simulink model "Model1"  (R2024b)
settings: Solver=ode8  StartTime=0.0  StopTime=simT  FixedStep=Ts  RelTol=1e-3
values from neighbouring files (symbols this model uses):
  C = 1    [HHparameters.m]
  EK = -12    [HHparameters.m]
  EL = 10.613    [HHparameters.m]
  ENa = 115    [HHparameters.m]
  gbar_K = 36    [HHparameters.m]
  gbar_Na = 120    [HHparameters.m]
  gL = 0.3    [HHparameters.m]
  minf0 = alpham0/(alpham0+betam0)    [HHparameters.m]
settings Model: LastModifiedBy=Matth

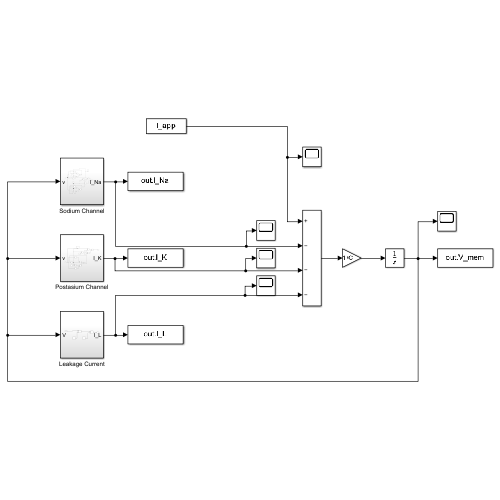
[thumbnail: Simulink's stored preview of the top-level diagram]
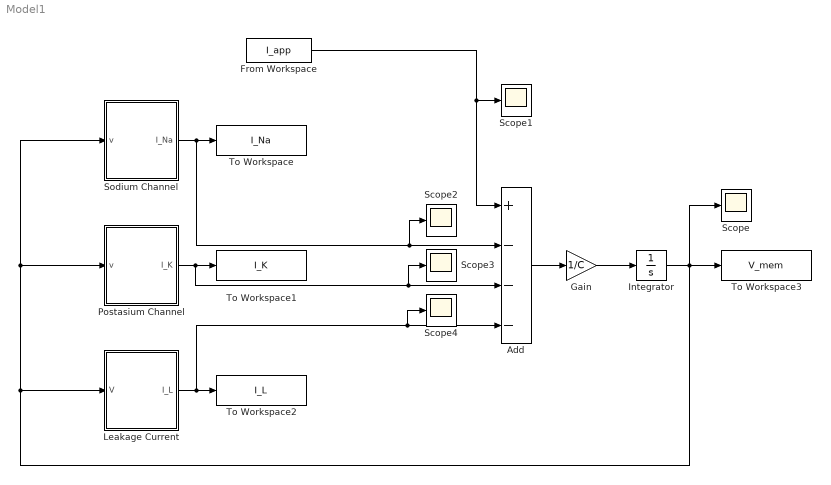
== system Model1 ==
  Add : Sum  Inputs=+---
  From Workspace : FromWorkspace  VariableName=I_app
  Gain : Gain  Gain=1/C
  Integrator : Integrator  InitialCondition=minf0
  Leakage Current : Subsystem
  Postasium Channel : Subsystem
  Scope{,1..4} (5 alike) : Scope
  Sodium Channel : Subsystem
  To Workspace : ToWorkspace  VariableName=I_Na  SampleTime=-1
  To Workspace1 : ToWorkspace  VariableName=I_K  SampleTime=-1
  To Workspace2 : ToWorkspace  VariableName=I_L  SampleTime=-1
  To Workspace3 : ToWorkspace  VariableName=V_mem  SampleTime=-1
  wires:
  Sodium Channel/1(I_Na) -> To Workspace/1, Scope2/1, Add/2
  Gain/1 -> Integrator/1
  Integrator/1 -> To Workspace3/1, Sodium Channel/1(v), Postasium Channel/1(v), Leakage Current/1(V), Scope/1
  Add/1 -> Gain/1
  Postasium Channel/1(I_K) -> To Workspace1/1, Add/3, Scope3/1
  Leakage Current/1(I_L) -> Scope4/1, Add/4, To Workspace2/1
  From Workspace/1 -> Scope1/1, Add/1

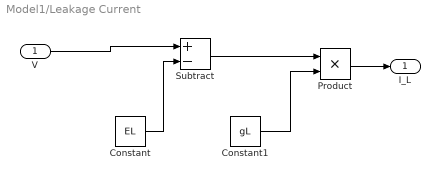
== system Model1/Leakage Current ==
  V : Inport
  Constant : Constant  Value=EL
  Constant1 : Constant  Value=gL
  Product : Product
  Subtract : Sum  Inputs=+-
  I_L : Outport
  wires:
  Constant1/1 -> Product/2
  Constant/1 -> Subtract/2
  V/1 -> Subtract/1
  Subtract/1 -> Product/1
  Product/1 -> I_L/1

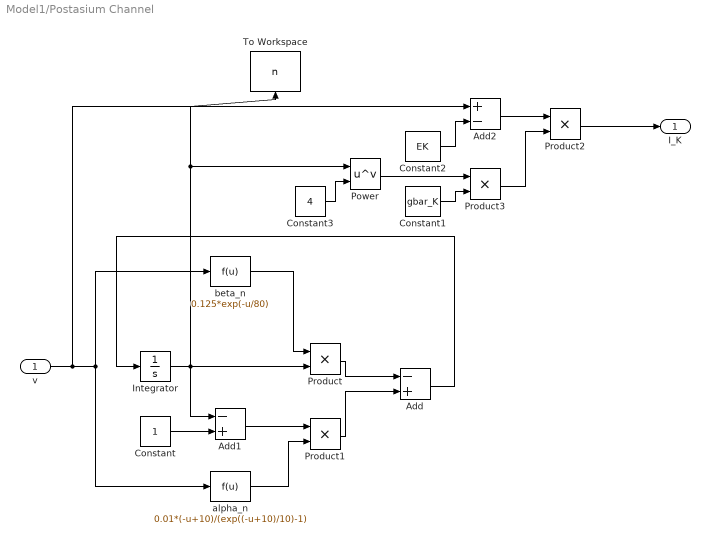
== system Model1/Postasium Channel ==
  v : Inport
  Add : Sum  Inputs=-+
  Add1 : Sum  Inputs=-+
  Add2 : Sum  Inputs=+-
  Constant : Constant
  Constant1 : Constant  Value=gbar_K
  Constant2 : Constant  Value=EK
  Constant3 : Constant  Value=4
  Integrator : Integrator  InitialCondition=0.1/(exp(1)-1)/(0.1/(exp(1)-1)+0.125)
  Power : Math  Operator=pow
  Product{,1..3} (4 alike) : Product
  To Workspace : ToWorkspace  VariableName=n  SaveFormat=Timeseries  SampleTime=-1
  alpha_n : Fcn  Expr=0.01*(-u+10)/(exp((-u+10)/10)-1)
  beta_n : Fcn  Expr=0.125*exp(-u/80)
  I_K : Outport
  wires:
  beta_n/1 -> Product/1
  Product/1 -> Add/1
  Product1/1 -> Add/2
  Add1/1 -> Product1/1
  Constant/1 -> Add1/2
  Add/1 -> Integrator/1
  Integrator/1 -> Product/2, Power/1, To Workspace/1, Add1/1
  Add2/1 -> Product2/1
  Product3/1 -> Product2/2
  Constant1/1 -> Product3/2
  Power/1 -> Product3/1
  Constant2/1 -> Add2/2
  Product2/1 -> I_K/1
  v/1 -> beta_n/1, alpha_n/1, Add2/1
  alpha_n/1 -> Product1/2
  Constant3/1 -> Power/2

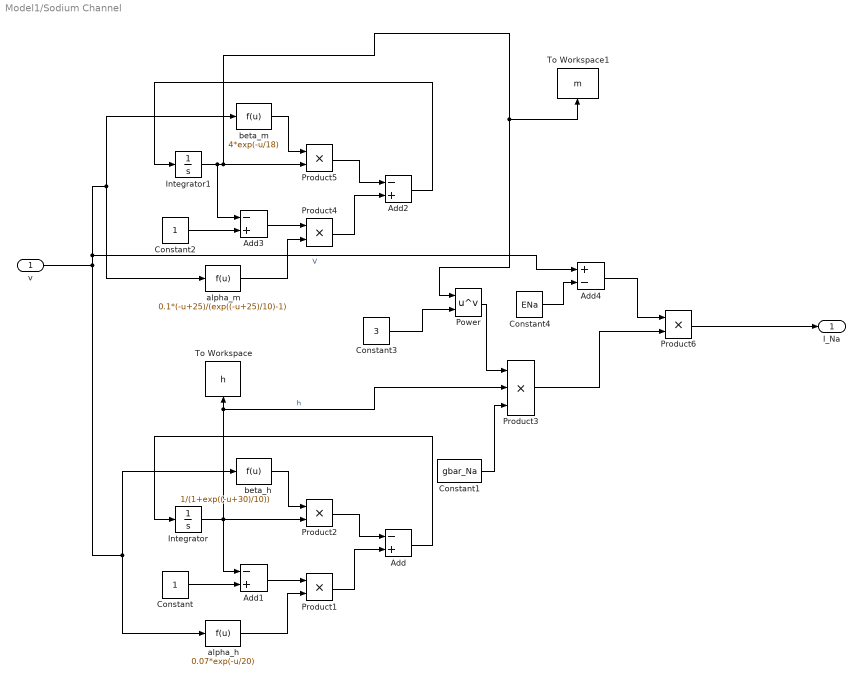
== system Model1/Sodium Channel ==
  v : Inport
  Add{,1..3} (4 alike) : Sum  Inputs=-+
  Add4 : Sum  Inputs=+-
  Constant : Constant
  Constant1 : Constant  Value=gbar_Na
  Constant2 : Constant
  Constant3 : Constant  Value=3
  Constant4 : Constant  Value=ENa
  Integrator : Integrator  InitialCondition=0.07/(0.07+1/(exp(3)+1))
  Integrator1 : Integrator  InitialCondition=2.5/(exp(2.5)-1)/(2.5/(exp(2.5)-1)+4)
  Power : Math  Operator=pow
  Product{1..2,4..6} (5 alike) : Product
  Product3 : Product  Inputs=3
  To Workspace : ToWorkspace  VariableName=h  SaveFormat=Timeseries  SampleTime=-1
  To Workspace1 : ToWorkspace  VariableName=m  SaveFormat=Timeseries  SampleTime=-1
  alpha_h : Fcn  Expr=0.07*exp(-u/20)
  alpha_m : Fcn  Expr=0.1*(-u+25)/(exp((-u+25)/10)-1)
  beta_h : Fcn  Expr=1/(1+exp((-u+30)/10))
  beta_m : Fcn  Expr=4*exp(-u/18)
  I_Na : Outport
  wires:
  Add1/1 -> Product1/1
  Product1/1 -> Add/2
  Constant/1 -> Add1/2
  alpha_h/1 -> Product1/2
  Product2/1 -> Add/1
  Integrator/1 -> Add1/1, Product3/2, To Workspace/1, Product2/2  "h"
  beta_h/1 -> Product2/1
  Add/1 -> Integrator/1
  Constant1/1 -> Product3/3
  beta_m/1 -> Product5/1
  alpha_m/1 -> Product4/2
  Product5/1 -> Add2/1
  Constant2/1 -> Add3/2
  Product4/1 -> Add2/2
  Add2/1 -> Integrator1/1
  Add3/1 -> Product4/1
  Integrator1/1 -> Power/1, To Workspace1/1, Product5/2, Add3/1
  v/1 -> Add4/1, alpha_m/1, beta_m/1, beta_h/1, alpha_h/1  "V"
  Power/1 -> Product3/1
  Constant4/1 -> Add4/2
  Add4/1 -> Product6/1
  Product3/1 -> Product6/2
  Product6/1 -> I_Na/1
  Constant3/1 -> Power/2
